simulink model "State_feedback_stabilizingcontroller"  (R2020b)
settings: Solver=FixedStepAuto  StartTime=0.0  StopTime=3  RelTol=1e-3
values from neighbouring files (symbols this model uses):
  D = [0]    [main.m]
settings Model: Creator=Kevin  LastModifiedBy=francesco

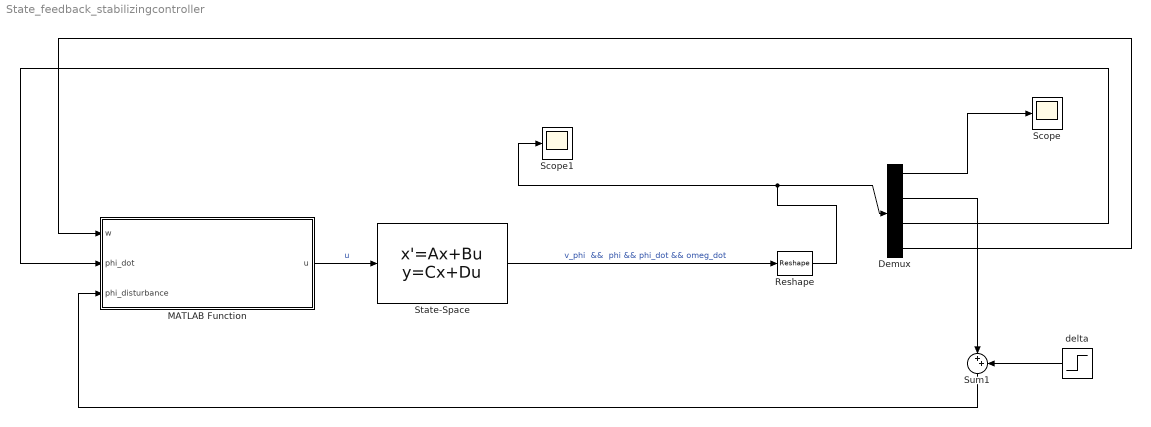
== system State_feedback_stabilizingcontroller ==
  Demux : Demux
  MATLAB Function : MATLAB Function  TreatAsAtomicUnit=on
  Reshape : Reshape  OutputDimensionality=Row vector (2-D)  OutputDimensions=[1,4]
  Scope : Scope
  Scope1 : Scope
  State-Space : StateSpace  A=[0 1 0; 23.5031 0 0.0045; -23.5031 0 -19.9513]  B=[0; 0.1393; -621.6819]  C=[107.47 0 0;1 0 0; 0 1 0; 0 0 1]  D=[0;0;0;0]  InitialCondition=[0.0019 0 0]
  Sum1 : Sum  Inputs=|++
  delta : Step  Time=1.5  Before=0.1  After=0.2  SampleTime=0
  wires:
  MATLAB Function/1(u) -> State-Space/1  "u"
  delta/1 -> Sum1/2
  State-Space/1 -> Reshape/1  "v_phi  &&  phi && phi_dot && omeg_dot"
  Demux/2 -> Sum1/1
  Reshape/1 -> Scope1/1, Demux/1
  Demux/3 -> MATLAB Function/2(phi_dot)
  Sum1/1 -> MATLAB Function/3(phi_disturbance)
  Demux/4 -> MATLAB Function/1(w)
  Demux/1 -> Scope/1

== matlab function State_feedback_stabilizingcontroller/MATLAB Function ==
  data: w input; u output; phi_dot input; phi_disturbance input
function u = state_feedback_control_law(w,phi_dot, phi_disturbance)

K=[2.29*10.^3 4.72*10.^2 0.08]
x=[w;phi_dot;phi_disturbance]

u = -K*x;
